simulink model "ECEF_to_LLA"  (R2016b)
settings: Solver=VariableStepAuto  StartTime=0.0  StopTime=10.0  RelTol=1e-3
undefined symbols (not defined in the file or in its folder): Earth, WGS84
libraries: aerolibtransform2 x1, aerolibgravity2 x1
settings Model: Creator=taylorreynolds  LastModifiedBy=taylorreynolds

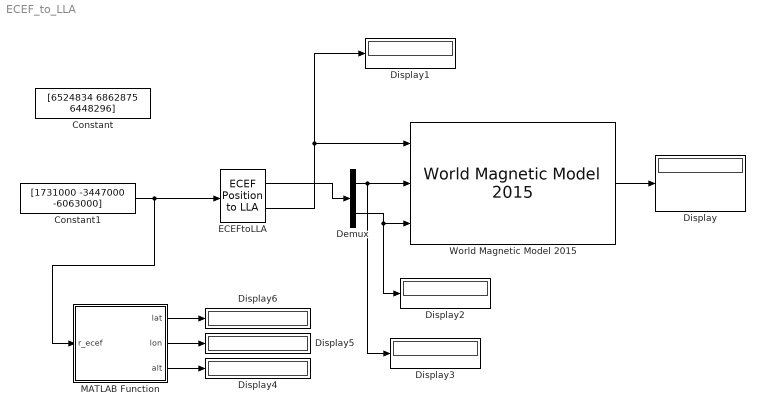
== system ECEF_to_LLA ==
  Constant : Constant  Value=[6524834 6862875 6448296]
  Constant1 : Constant  Value=[1731000 -3447000 -6063000]
  Demux : Demux  Outputs=2
  Display{,1..6} (7 alike) : Display
  ECEFtoLLA : aerolibtransform2/ECEF Position to LLA  units=Metric (MKS)  ptype=Earth (WGS84)  F=1/298.257223563  R=6378137
  MATLAB Function : MATLAB Function  TreatAsAtomicUnit=on
  World Magnetic Model 2015 : aerolibgravity2/World Magnetic Model 2015  units=Metric (MKS)  time_in=off  month=October  day=19  year=2017  action=Warning  h_out=off  dec_out=off  inc_out=off  ti_out=off
  wires:
  Demux/2 -> Display2/1, World Magnetic Model 2015/3
  Demux/1 -> Display3/1, World Magnetic Model 2015/2
  ECEFtoLLA/1 -> Demux/1
  ECEFtoLLA/2 -> World Magnetic Model 2015/1, Display1/1
  Constant1/1 -> MATLAB Function/1(r_ecef), ECEFtoLLA/1
  World Magnetic Model 2015/1 -> Display/1
  MATLAB Function/3(alt) -> Display4/1
  MATLAB Function/1(lat) -> Display6/1
  MATLAB Function/2(lon) -> Display5/1

== matlab function ECEF_to_LLA/MATLAB Function ==
  data: r_ecef input size=3; lat output size=1; lon output size=1; alt output size=1
% ECEF2LLA - convert earth-centered earth-fixed (ECEF)
%            cartesian coordinates to latitude, longitude,
%            and altitude
%
% USAGE:
% [lat,lon,alt] = ecef2lla(x,y,z)
%
% lat = geodetic latitude (radians)
% lon = longitude (radians)
% alt = height above WGS84 ellipsoid (m)
% x = ECEF X-coordinate (m)
% y = ECEF Y-coordinate (m)
% z = ECEF Z-coordinate (m)
%
% HuskySat-1, ADCS Subsystem
% Last Updated: T. Reynolds - 10.18.17


function [lat,lon,alt] = ecef2lla(r_ecef)

rI   = r_ecef(1);
rJ   = r_ecef(2);
rZ   = r_ecef(3);

% WGS84 ellipsoid constants:
RAD2DEG     = 180/pi;
RE = 6378137;
EE = 8.1819190842622e-2;
EE2     = EE^2;

r           = norm(r_ecef);
r_d_sat     = sqrt(rI^2+rJ^2);
sind_a       = rJ/r_d_sat;
cosd_a       = rI/r_d_sat;
% compute longitude
lons        = asind(sind_a);
lonc        = acosd(cosd_a);
lon         = 0.5*(lons+lonc);

tan_d       = rZ/r_d_sat;

lat         = atand(tan_d);
r_d         = r_d_sat;
r_z         = rZ;
lat_old     = 1e3;
iter_max    = 20;
iter        = 0;
CE          = 0;
while( (abs(lat-lat_old) > 1e-4) && iter < iter_max )
    CE          = RE/(sqrt(1-EE2*(sind(lat)^2)));
    tan_d       = (r_z + CE*EE2*sind(lat))/r_d;
    lat_old     = lat;
    lat         = atand(tan_d);
    iter        = iter + 1;
end

h_ellp      = r_d/(cosd(lat)) - CE;

if( lat <= 0.0175 )
    SE      = RE*(1-EE2)/(sqrt(1-EE2*(sind(lat)^2)));
    h_ellp  = r_z/(sind(lat)) - SE;
end

alt     = h_ellp;

return
